simulink model "Driver_PwtrBlkset_V1"  (R2018a)
settings: Solver=ode45  StartTime=0.0  StopTime=660  FixedStep=0.001  EnableMultiTasking=on
PreLoadFcn:
  | Driver_PreLoad
undefined symbols (not defined in the file): sigbuilder_block
libraries: autolibshared x1, simulink x1
settings Model: Creator=Nishito  LastModifiedBy=nishito
settings SolverCC: MaxOrder=2  ZeroCrossControl=DisableAll
settings DataIOCC: SaveFormat=Array  SignalLoggingSaveFormat=ModelDataLogs  SaveOutput=off  SignalLogging=off  DSMLogging=off  SaveTime=off
settings OptimizationCC: ExpressionDepthLimit=2147483647  LifeSpan=inf
settings DebuggingCC: AlgebraicLoopMsg=error  UnderspecifiedInitializationDetection=Classic  MergeDetectMultiDrivingBlocksExec=none  FcnCallInpInsideContextMsg=warning  StateNameClashWarn=warning  SFUnexpectedBacktrackingDiag=warning  SFNoUnconditionalDefaultTransitionDiag=warning  SFExecutionAtInitializationDiag=none
settings HardwareCC: ProdBitPerPointer=32  ProdBitPerSizeT=32  ProdBitPerPtrDiffT=32  ProdLargestAtomicFloat=None  ProdIntDivRoundTo=Undefined  ProdEndianess=Unspecified  ProdWordSize=32  ProdHWDeviceType=32-bit Generic
settings ModelReferenceCC: PropagateSignalLabelsOutOfModel=off
settings CodeAppCC: StateflowObjectComments=on
settings GRTTargetCC: TargetLangStandard=C89/C90 (ANSI)  GeneratePreprocessorConditionals=Disable all  CombineOutputUpdateFcns=off  GRTInterface=on
settings ConfigComp: CovMetricSettings=dw  CovHtmlReporting=on  CovSaveCumulativeToWorkspaceVar=on  CovSaveSingleToWorkspaceVar=on  CovExternalEMLEnable=off  CovSFcnEnable=off
settings SimscapeCC: SimscapeNormalizeSystem=off  SimscapeLogSimulationStatistics=on  SimscapeLogOpenViewer=on  SimscapeLogLimitData=off

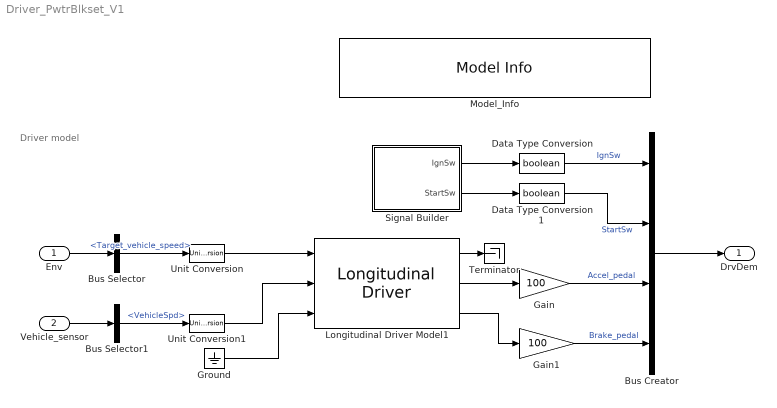
== system Driver_PwtrBlkset_V1 ==
  note: Driver model
  Env : Inport  OutDataTypeStr=Bus: Environment_Bus
      settings: AttributesFormatString=%<OutDataTypeStr>
  Vehicle_sensor : Inport  Port=2  OutDataTypeStr=Bus: Vehicle_sensor_Bus
      settings: AttributesFormatString=%<OutDataTypeStr>
  Bus Creator : BusCreator  Inputs=4  OutDataTypeStr=Bus: Driver_demand_Bus
      settings: AttributesFormatString=%<OutDataTypeStr>
  Bus Selector : BusSelector  OutputSignals=Target_vehicle_speed
  Bus Selector1 : BusSelector  OutputSignals=Brake_sensor.VehicleSpd
  Data Type Conversion : DataTypeConversion  OutDataTypeStr=boolean
  Data Type Conversion1 : DataTypeConversion  OutDataTypeStr=boolean
  Gain : Gain  Gain=100
  Gain1 : Gain  Gain=100
  Ground : Ground
  Longitudinal Driver Model1 : autolibshared/Longitudinal Driver  aMode=aMode  vnom=5  Kp=1  Ki=0.2  Kaw=1  Kff=.1  Kg=0  tauerr=0.01
      settings: SourceProductName=Powertrain Blockset  SourceProductBaseCode=PW
  Model_Info : simulink/Model-Wide Utilities/Model Info  Frame=on  DisplayStringWithTags=|  HorizontalTextAlignment=Left  LeftAlignmentValue=0.02
      | Version  %<ModelVersion>
      | LastModifided by %<LastModifiedBy>  Date %<LastModificationDate>
      | Description  %<Description>
  Signal Builder : Subsystem  Tag=STV Subsys  LoadFcn=sigbuilder_block('load');  StartFcn=sigbuilder_block('start');  StopFcn=sigbuilder_block('stop');  ClipboardFcn=sigbuilder_block('clipboard');  mask(Sigbuilder block){tuvar=[0:10]}
      mask help: Simulink:masks:SigbuilderBlock_MD
      mask init:
      | if ~strcmp(get_param(bdroot(gcbh),'SimulationStatus'),'stopped') tuvar = sigbuilder_block('maskInit'); end
      settings: CopyFcn=sigbuilder_block('copy');  DeleteFcn=sigbuilder_block('delete');  ModelCloseFcn=sigbuilder_block('modelClose');  PreSaveFcn=sigbuilder_block('preSave');  PauseFcn=sigbuilder_block('pause');  ContinueFcn=sigbuilder_block('continue');  NameChangeFcn=sigbuilder_block('namechange');  OpenFcn=sigbuilder_block('open',[0 33 1020 493.5 ]);  CloseFcn=sigbuilder_block('close');
      mask Display: plot(0, 0, 100, 100,[2, 2, 32, 32, 2], [68, 8, 8, 68, 68],[32, 2], [38, 38], [32, 19, 2],[53, 60, 44], [32, 17, 17, 2],[16, 16, 31, 31]);txt = getActiveGroup(gcbh);text(2, 100, txt,'verticalAlignment', 'top');
  Terminator : Terminator
  Unit Conversion : UnitConversion
  Unit Conversion1 : UnitConversion
  DrvDem : Outport  OutDataTypeStr=Bus: Driver_demand_Bus
      settings: AttributesFormatString=%<OutDataTypeStr>
  wires:
  Bus Creator/1 -> DrvDem/1
  Gain/1 -> Bus Creator/3  "Accel_pedal"
  Gain1/1 -> Bus Creator/4  "Brake_pedal"
  Env/1 -> Bus Selector/1
  Vehicle_sensor/1 -> Bus Selector1/1
  Bus Selector1/1 -> Unit Conversion1/1  "<VehicleSpd>"
  Bus Selector/1 -> Unit Conversion/1  "<Target_vehicle_speed>"
  Longitudinal Driver Model1/2 -> Gain/1
  Longitudinal Driver Model1/3 -> Gain1/1
  Ground/1 -> Longitudinal Driver Model1/3
  Longitudinal Driver Model1/1 -> Terminator/1
  Data Type Conversion/1 -> Bus Creator/1  "IgnSw"
  Data Type Conversion1/1 -> Bus Creator/2  "StartSw"
  Signal Builder/1(IgnSw) -> Data Type Conversion/1
  Signal Builder/2(StartSw) -> Data Type Conversion1/1
  Unit Conversion/1 -> Longitudinal Driver Model1/1
  Unit Conversion1/1 -> Longitudinal Driver Model1/2

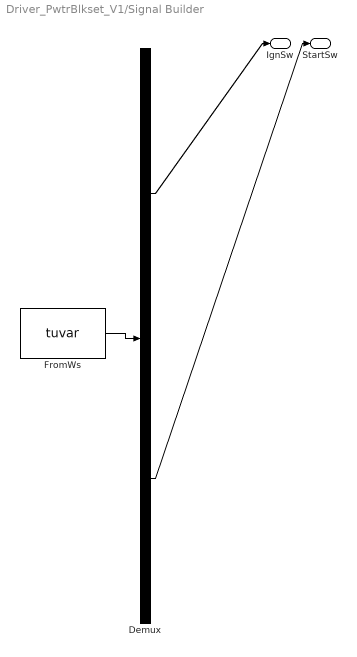
== system Driver_PwtrBlkset_V1/Signal Builder ==
  Demux : Demux  Tag=STV Demux  Outputs=2
  FromWs : FromWorkspace  Tag=STV FromWs  VariableName=tuvar  SampleTime=0
      SigBuilderData=|
      | common.afterFinalStr = 'Extrapolate'
      | common.sampleTime = 0
      | dataSet.timeRange = [0 10]
      | dataSet.name = 'Group 1'
      | sbobj.Groups.Name = 'Group 1'
      | sbobj.Groups.Signals(1).Name = 'IgnSw'
      | sbobj.Groups.Signals(1).XData = [0 0.5 0.5 10]
      | sbobj.Groups.Signals(1).YData = [0 0 1 1]
      | sbobj.Groups.Signals(2).Name = 'StartSw'
      | sbobj.Groups.Signals(2).XData = [0 1 1 2 2 10]
      | sbobj.Groups.Signals(2).YData = [0 0 1 1 0 0]
  IgnSw : Outport  Tag=STV Outport
  StartSw : Outport  Tag=STV Outport  Port=2
  wires:
  FromWs/1 -> Demux/1
  Demux/1 -> IgnSw/1
  Demux/2 -> StartSw/1
